simulink model "WT_besser"  (R2023a)
settings: Solver=VariableStepAuto  StartTime=0.0  StopTime=inf  RelTol=1e-3
undefined symbols (not defined in the file or in its folder): National_Instruments, PCI
libraries: sldrtlib x3
settings Model: Creator=EAL  LastModifiedBy=EAL

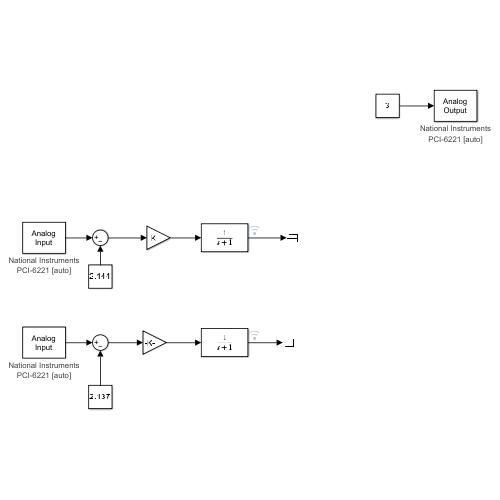
[thumbnail: Simulink's stored preview of the top-level diagram]
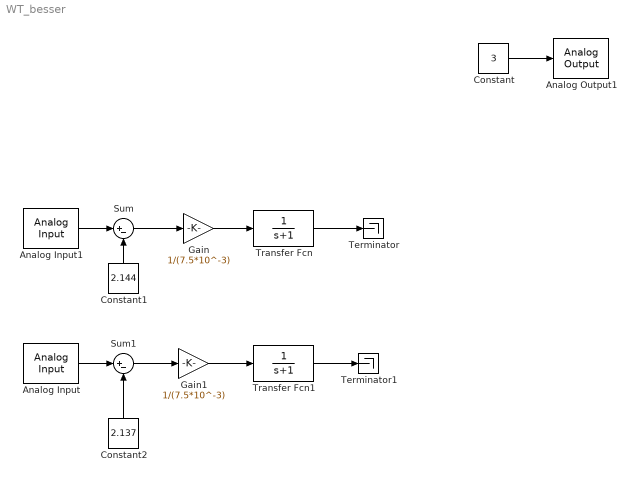
== system WT_besser ==
  Analog Input : sldrtlib/Analog Input  SampleTime=0.1  MaxMissedTicks=10  ShowMissedTicks=off  YieldWhenWaiting=off  DrvName=National_Instruments/PCI-6221  DrvAddress=4294967295  DrvOptions=[0 0 0 0 0]  Channels=2  RangeMode=1  VoltRange=1  DataType=1
      settings: AttributesFormatString=National Instruments\nPCI-6221 [auto]
  Analog Input1 : sldrtlib/Analog Input  SampleTime=0.1  MaxMissedTicks=10  ShowMissedTicks=off  YieldWhenWaiting=off  DrvName=National_Instruments/PCI-6221  DrvAddress=4294967295  DrvOptions=[0 0 0 0 0]  Channels=1  RangeMode=1  VoltRange=1  DataType=1
      settings: AttributesFormatString=National Instruments\nPCI-6221 [auto]
  Analog Output1 : sldrtlib/Analog Output  SampleTime=0.1  MaxMissedTicks=10  ShowMissedTicks=off  YieldWhenWaiting=off  DrvName=National_Instruments/PCI-6221  DrvAddress=4294967295  DrvOptions=[0 0 0 0 0]  Channels=1  RangeMode=1  VoltRange=1  InitialValue=[]  FinalValue=[]
      settings: AttributesFormatString=National Instruments\nPCI-6221 [auto]
  Constant : Constant  Value=3
  Constant1 : Constant  Value=2.144
  Constant2 : Constant  Value=2.137
  Gain : Gain  Gain=1/(7.5*10^-3)
  Gain1 : Gain  Gain=1/(7.5*10^-3)
  Sum : Sum  Inputs=|+-
  Sum1 : Sum  Inputs=|+-
  Terminator : Terminator
  Terminator1 : Terminator
  Transfer Fcn : TransferFcn  Denominator=[1 1]
  Transfer Fcn1 : TransferFcn  Denominator=[1 1]
  wires:
  Constant/1 -> Analog Output1/1
  Transfer Fcn/1 -> Terminator/1
  Transfer Fcn1/1 -> Terminator1/1
  Gain/1 -> Transfer Fcn/1
  Gain1/1 -> Transfer Fcn1/1
  Analog Input1/1 -> Sum/1
  Sum/1 -> Gain/1
  Constant1/1 -> Sum/2
  Analog Input/1 -> Sum1/1
  Sum1/1 -> Gain1/1
  Constant2/1 -> Sum1/2
